simulink model "North_Country_Grid_2024a"  (R2024a)
settings: Solver=VariableStepAuto  StartTime=0.0  StopTime=10  RelTol=1e-3
PreLoadFcn:
  | Ts=50e-6;
InitFcn:
  | xInitial = WindFarmType4AverageModelInit;
  | Ts=50e-6;
undefined symbols (not defined in the file or in its folder): D1, D11, Delta, DiscIntNeverNeededParam, find_system, Fnom_I, Fnom_R, Idc_nom, lagging, level, pulse, test_alpha, Vdc_nom, VLL_nom_I, VLL_nom_R
libraries: spsSecondOrderFilterLib x47, powerlib_extras x38, simulink x34, spsThreePhaseVIMeasurementLib x30, spsFirstOrderFilterLib x29, simulink_extras x26, spsabctodq0Lib x25, spsThreePhaseTransformerTwoWindingsLib x19, spsThreePhaseBreakerLib x18, spsThreePhasePISectionLineLib x17, spsControlledVoltageSourceLib x15, spsOnDelayLib x12
(part 1 of 18)
settings Model: FPTRunName=Active  Creator=The MathWorks, Inc.  LastModifiedBy=prankfarsons
settings DebuggingCC: UnderspecifiedInitializationDetection=Classic  MergeDetectMultiDrivingBlocksExec=none
settings ModelReferenceCC: PropagateSignalLabelsOutOfModel=off

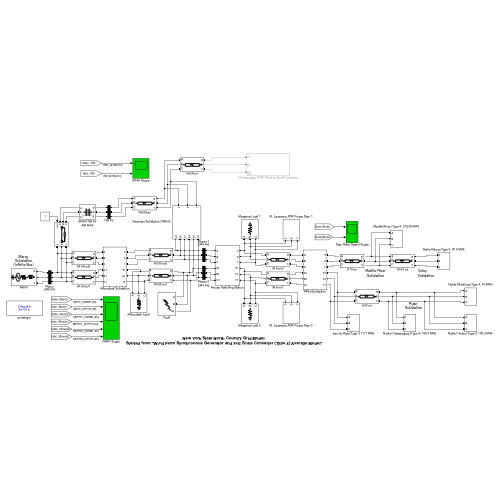
[thumbnail: Simulink's stored preview of the top-level diagram]
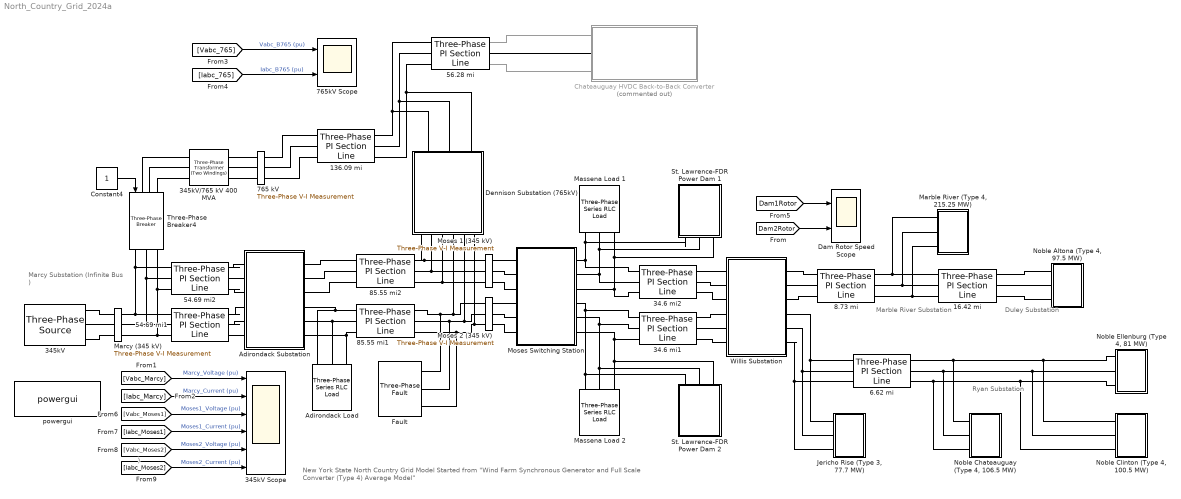
== system North_Country_Grid_2024a ==
  note: )
  note: Marcy Substation
      | (Infinite Bus )
  note: Ryan Substation
  note: New York State North Country Grid Model
      | Started from "Wind Farm Synchronous Generator and Full Scale Converter (Type 4) Average Model"
  note: Marble River Substation
  note: Duley Substation
  " Dam Rotor Speed Scope" : Scope  NumInputPorts=2
  136.09 mi : spsThreePhasePISectionLineLib/Three-Phase PI Section Line  LConnTagsString=a|b|c  RConnTagsString=A|B|C  Length=219.015  Frequency=60  Resistances=[0.0117 0.3864]  Inductances="[9.44e-4  4.1264e-3]"  Capacitances=[4e-10 7.751e-9]
  16.42 mi : spsThreePhasePISectionLineLib/Three-Phase PI Section Line  LConnTagsString=a|b|c  RConnTagsString=A|B|C  Length=26.425  Frequency=60  Resistances=[ 0.0283 0.3864]  Inductances="[ 1.146e-3  4.1264e-3]"  Capacitances=[20.9e-9 7.751e-9]
  34.6 mi1 : spsThreePhasePISectionLineLib/Three-Phase PI Section Line  LConnTagsString=a|b|c  RConnTagsString=A|B|C  Length=55.68  Frequency=60  Resistances=[ 0.0283 0.3864]  Inductances="[ 1.146e-3  4.1264e-3]"  Capacitances=[20.9e-9 7.751e-9]
  34.6 mi2 : spsThreePhasePISectionLineLib/Three-Phase PI Section Line  LConnTagsString=a|b|c  RConnTagsString=A|B|C  Length=55.68  Frequency=60  Resistances=[ 0.0283 0.3864]  Inductances="[ 1.146e-3  4.1264e-3]"  Capacitances=[20.9e-9 7.751e-9]
  345kV : spsThreePhaseSourceLib/Three-Phase Source  InternalConnection=Yg  VoltagePhases=off  Voltage=(345000)*0.996321  PhaseAngle=0.044565  Voltage_phases=[25e3 25e3 25e3]/sqrt(3)  PhaseAngles_phases=[0 -120 +120]  Frequency=60  NonIdealSource=on  SpecifyImpedance=off  Resistance=0.8929  Inductance=16.58e-3  ShortCircuitLevel=100e6  BaseVoltage=345e3  XRratio=7  BusType=swing  Pref=100000000  Qref=0  Prefabc=[10e3, 10e3, 10e3]  Qrefabc=[0, 0, 0]  Qmin=-Inf  Qmax=Inf
  345kV Scope : Scope  NumInputPorts=6
  345kV/765 kV 400 MVA : spsThreePhaseTransformerTwoWindingsLib/Three-Phase Transformer (Two Windings)  Winding1Connection=Delta (D11)  Winding2Connection=Yg  CoreType=Three single-phase transformers  SetSaturation=off  Hysteresis=off  DataFile='basic_model'  SetInitialFlux=off  Measurements=None  UNITS=pu  NominalPower=[400e6 60 ]  Winding1="[ 345e3  0.0125   0.025 ]"  Winding2="[765e3  0.0125   0.025]"  Rm=500  Lm=inf  L0=0.5  Saturation="[ 0,0  ;  0.005,1.2  ;  1.0,1.4 ]"  InitialFluxes=[ 0.8 , -0.8 , 0.7 ]  BreakLoop=off  DiscreteSolver=Trapezoidal iterative  DataType=off  TransfoNumber=0
  54.69 mi1 : spsThreePhasePISectionLineLib/Three-Phase PI Section Line  LConnTagsString=a|b|c  RConnTagsString=A|B|C  Length=88.015  Frequency=60  Resistances=[ 0.0283 0.3864]  Inductances="[ 1.146e-3  4.1264e-3]"  Capacitances=[20.9e-9 7.751e-9]
  54.69 mi2 : spsThreePhasePISectionLineLib/Three-Phase PI Section Line  LConnTagsString=a|b|c  RConnTagsString=A|B|C  Length=88.015  Frequency=60  Resistances=[ 0.0283 0.3864]  Inductances="[ 1.146e-3  4.1264e-3]"  Capacitances=[20.9e-9 7.751e-9]
  56.28 mi : spsThreePhasePISectionLineLib/Three-Phase PI Section Line  LConnTagsString=a|b|c  RConnTagsString=A|B|C  Length=90.57  Frequency=60  Resistances=[0.0117 0.3864]  Inductances="[9.44e-4  4.1264e-3]"  Capacitances=[4e-10 7.751e-9]
  6.62 mi : spsThreePhasePISectionLineLib/Three-Phase PI Section Line  LConnTagsString=a|b|c  RConnTagsString=A|B|C  Length=10.654  Frequency=60  Resistances=[ 0.0283 0.3864]  Inductances="[ 1.146e-3  4.1264e-3]"  Capacitances=[20.9e-9 7.751e-9]
  765 kV : spsThreePhaseVIMeasurementLib/Three-Phase V-I Measurement  VoltageMeasurement=phase-to-ground  SetLabelV=on  LabelV=Vabc_765  Vpu=on  VpuLL=off  CurrentMeasurement=yes  SetLabelI=on  LabelI=Iabc_765  Ipu=on  Pbase=1590.45e6  Vbase=765e3  OutputType=Complex  PhasorSimulation=off  PSBequivalent=0
  765kV Scope : Scope  NumInputPorts=2
  8.73 mi : spsThreePhasePISectionLineLib/Three-Phase PI Section Line  LConnTagsString=a|b|c  RConnTagsString=A|B|C  Length=14.049  Frequency=60  Resistances=[ 0.0283 0.3864]  Inductances="[ 1.146e-3  4.1264e-3]"  Capacitances=[20.9e-9 7.751e-9]
  85.55 mi1 : spsThreePhasePISectionLineLib/Three-Phase PI Section Line  LConnTagsString=a|b|c  RConnTagsString=A|B|C  Length=137.679  Frequency=60  Resistances=[ 0.0283 0.3864]  Inductances="[ 1.146e-3  4.1264e-3]"  Capacitances=[20.9e-9 7.751e-9]
  85.55 mi2 : spsThreePhasePISectionLineLib/Three-Phase PI Section Line  LConnTagsString=a|b|c  RConnTagsString=A|B|C  Length=137.679  Frequency=60  Resistances=[ 0.0283 0.3864]  Inductances="[ 1.146e-3  4.1264e-3]"  Capacitances=[20.9e-9 7.751e-9]
  Adirondack Load : spsThreePhaseSeriesRLCLoadLib/Three-Phase Series RLC Load  LConnTagsString=A|B|C  Configuration=Y (grounded)  NominalVoltage=345e3  Vabc=[1e3 1e3 1e3]  Vabcp=[1e3 1e3 1e3]  NominalFrequency=60  UnbalancedPower=off  ActivePower=100000000  InductivePower=0  CapacitivePower=0  Pabc=[10e3 9e3 11e3]  QLabc=[100 90 110]  QCabc=[100 90 110]  Pabcp=[10e3 9e3 11e3]  QLabcp=[100 90 110]  QCabcp=[100 90 110]  Measurements=None  LoadType=constant Z
  Adirondack Substation : Subsystem
  Chateauguay HVDC Back-to-Back Converter : Subsystem  Commented=on
  Constant4 : Constant
  Dennison Substation (765kV) : Subsystem
      settings: PortSchema="{\"entries\":[{\"content\":{\"sides\":[{\"content\":{},\"type\":\"ConnectorPlacement.EquallySpacedRectSide\",\"uuid\":\"bf43bd2c-e3a2-40b5-9bf7-800fca43b76b\"},{\"content\":{\"side\":\"RIGHT\"},\"type\":\"ConnectorPlacement.EquallySpacedRectSide\",\"uuid\":\"0e930517-6b8c-4af0-8fde-37d9fd24c178\"},{\"content\":{\"connectorIds\":[\"LConn1\",\"LConn2\",\"LConn3\"],\"side\":\"TOP\"},\"type\":\"ConnectorPlacement.EquallySpacedRectSide\",\"uuid\":\"782c9b1f-adb6-4d18-a320-946579c28cc2\"},{\"content\":{\"connectorIds\":[\"RConn1\",\"RConn2\",\"RConn3\",\"RConn4\",\"RConn5\",\"RConn6\"],\"side\":\"BOTTOM\"},\"type\":\"ConnectorPlacement.EquallySpacedRectSide\",\"uuid\":\"c85884d3-7f69-4181-84c4-a6d381e135a3\"}]},\"type\":\"ConnectorPlacement.EquallySpacedConnector\",\"uuid\":\"dcc53c74-8f9c-434c-bbfe-404556b3529c\"}],\"packageUris\":[\"http://schema.mathworks.com/mf0/Connector/R2020b\"],\"version\":\"1.0\"}"
  Fault : spsThreePhaseFaultLib/Three-Phase Fault  InitialStates=0  FaultA=on  FaultB=on  FaultC=on  GroundFault=on  SwitchTimes="[4  4.3]"  External=off  SwitchStatus=NaN  FaultResistance=0.001  GroundResistance=0.01  SnubberResistance=1e6  SnubberCapacitance=inf  Measurements=None
  "Jericho Rise (Type 3, 77.7 MW)" : Subsystem
  "Marble River (Type 4, 215.25 MW)" : Subsystem
  Marcy (345 kV) : spsThreePhaseVIMeasurementLib/Three-Phase V-I Measurement  VoltageMeasurement=phase-to-ground  SetLabelV=on  LabelV=Vabc_Marcy  Vpu=on  VpuLL=off  CurrentMeasurement=yes  SetLabelI=on  LabelI=Iabc_Marcy  Ipu=on  Pbase=648.45e6  Vbase=345e3  OutputType=Complex  PhasorSimulation=off  PSBequivalent=0
  Massena Load 1 : spsThreePhaseSeriesRLCLoadLib/Three-Phase Series RLC Load  LConnTagsString=A|B|C  Configuration=Y (grounded)  NominalVoltage=345e3  Vabc=[1e3 1e3 1e3]  Vabcp=[1e3 1e3 1e3]  NominalFrequency=60  UnbalancedPower=off  ActivePower=150000000  InductivePower=0  CapacitivePower=0  Pabc=[10e3 9e3 11e3]  QLabc=[100 90 110]  QCabc=[100 90 110]  Pabcp=[10e3 9e3 11e3]  QLabcp=[100 90 110]  QCabcp=[100 90 110]  Measurements=None  LoadType=constant Z
  Massena Load 2 : spsThreePhaseSeriesRLCLoadLib/Three-Phase Series RLC Load  LConnTagsString=A|B|C  Configuration=Y (grounded)  NominalVoltage=345e3  Vabc=[1e3 1e3 1e3]  Vabcp=[1e3 1e3 1e3]  NominalFrequency=60  UnbalancedPower=off  ActivePower=150000000  InductivePower=0  CapacitivePower=0  Pabc=[10e3 9e3 11e3]  QLabc=[100 90 110]  QCabc=[100 90 110]  Pabcp=[10e3 9e3 11e3]  QLabcp=[100 90 110]  QCabcp=[100 90 110]  Measurements=None  LoadType=constant Z
  Moses 1 (345 kV) : spsThreePhaseVIMeasurementLib/Three-Phase V-I Measurement  VoltageMeasurement=phase-to-ground  SetLabelV=on  LabelV=Vabc_Moses1  Vpu=on  VpuLL=off  CurrentMeasurement=yes  SetLabelI=on  LabelI=Iabc_Moses1  Ipu=on  Pbase=648.45e6  Vbase=345e3  OutputType=Complex  PhasorSimulation=off  PSBequivalent=0
  Moses 2 (345 kV) : spsThreePhaseVIMeasurementLib/Three-Phase V-I Measurement  VoltageMeasurement=phase-to-ground  SetLabelV=on  LabelV=Vabc_Moses2  Vpu=on  VpuLL=off  CurrentMeasurement=yes  SetLabelI=on  LabelI=Iabc_Moses2  Ipu=on  Pbase=648.45e6  Vbase=345e3  OutputType=Complex  PhasorSimulation=off  PSBequivalent=0
  Moses Switching Station : Subsystem
  "Noble Altona (Type 4, 97.5 MW)" : Subsystem
  "Noble Chateauguay (Type 4, 106.5 MW)" : Subsystem
  "Noble Clinton (Type 4, 100.5 MW)" : Subsystem
  "Noble Ellenburg (Type 4, 81 MW)" : Subsystem
  St. Lawrence-FDR Power Dam 1 : Subsystem
  St. Lawrence-FDR Power Dam 2 : Subsystem
  Three-Phase Breaker4 : spsThreePhaseBreakerLib/Three-Phase Breaker  InitialState=closed  SwitchA=on  SwitchB=on  SwitchC=on  SwitchTimes="[1/60  5/60]"  External=on  BreakerResistance=0.01  SnubberResistance=1e6  SnubberCapacitance=inf  Measurements=None
  Willis Substation : Subsystem
  powergui : spspowerguiLib/powergui  SimulationMode=Discrete  SampleTime=Ts  frequency=60  Iterations=50  frequencyindice=0  Pbase=100e6  ErrMax=1e-4  UnitsV=kV  UnitsW=MW  buscounter=0  FunctionMessages=off  echomessages=off  EnableUseOfTLC=off  CurrentSourceSwitches=off  DisableSnubberDevices=off  DisableRonSwitches=off  DisableVfSwitches=off  DisplayEquations=off  AutomaticDiscreteSolvers=off  SolverType=Tustin/Backward Euler (TBE)  Interpol=off  ExternalGateDelay=off  methode=off  Ts=0  x0status=blocks  SPID=off  SwTol=0  HookPort=off  NonlinearTolerance=1e-4  nMaxIteration=100  ContinueOnMaxIteration=off  RestoreLinks=warning  ResistiveCurrentMeasurement=off  Frange=[0:2:500]  Ylog=off  Xlog=on  ShowGrid=off  save=off  variable=ZData  structure=0  ZoomFFT=on  StartTime=0.0  cycles=1  DisplayStyle=1  fundamental=60  FreqAxis=off  MaxFrequency=1000  frequencyindicesteady=1  RmsSteady=1  display=off
  wires:
  [Vabc_Marcy] -> 345kV Scope/1  "Marcy_Voltage (pu)"
  [Iabc_Marcy] -> 345kV Scope/2  "Marcy_Current (pu)"
  Constant4/1 -> Three-Phase Breaker4/1
  [Vabc_765] -> 765kV Scope/1  "Vabc_B765 (pu)"
  [Iabc_765] -> 765kV Scope/2  "Iabc_B765 (pu)"
  [Dam2Rotor] -> " Dam Rotor Speed Scope"/2
  [Dam1Rotor] -> " Dam Rotor Speed Scope"/1
  [Vabc_Moses1] -> 345kV Scope/3  "Moses1_Voltage (pu)"
  [Iabc_Moses1] -> 345kV Scope/4  "Moses1_Current (pu)"
  [Vabc_Moses2] -> 345kV Scope/5  "Moses2_Voltage (pu)"
  [Iabc_Moses2] -> 345kV Scope/6  "Moses2_Current (pu)"
  connections:
  16.42 mi/RConn1 -- "Noble Altona (Type 4, 97.5 MW)"/LConn1
  16.42 mi/RConn2 -- "Noble Altona (Type 4, 97.5 MW)"/LConn2
  16.42 mi/RConn3 -- "Noble Altona (Type 4, 97.5 MW)"/LConn3
  8.73 mi/RConn1 -- "Marble River (Type 4, 215.25 MW)"/LConn1 -- 16.42 mi/LConn1
  8.73 mi/RConn2 -- "Marble River (Type 4, 215.25 MW)"/LConn2 -- 16.42 mi/LConn2
  8.73 mi/RConn3 -- "Marble River (Type 4, 215.25 MW)"/LConn3 -- 16.42 mi/LConn3
  "Noble Chateauguay (Type 4, 106.5 MW)"/LConn1 -- 6.62 mi/RConn1 -- "Noble Ellenburg (Type 4, 81 MW)"/LConn1 -- "Noble Clinton (Type 4, 100.5 MW)"/LConn1
  "Noble Chateauguay (Type 4, 106.5 MW)"/LConn2 -- 6.62 mi/RConn2 -- "Noble Ellenburg (Type 4, 81 MW)"/LConn2 -- "Noble Clinton (Type 4, 100.5 MW)"/LConn2
  "Noble Chateauguay (Type 4, 106.5 MW)"/LConn3 -- 6.62 mi/RConn3 -- "Noble Ellenburg (Type 4, 81 MW)"/LConn3 -- "Noble Clinton (Type 4, 100.5 MW)"/LConn3
  Marcy (345 kV)/RConn1 -- Three-Phase Breaker4/RConn1 -- 54.69 mi2/LConn1 -- 54.69 mi1/LConn1
  Marcy (345 kV)/RConn2 -- Three-Phase Breaker4/RConn2 -- 54.69 mi2/LConn2 -- 54.69 mi1/LConn2
  Marcy (345 kV)/RConn3 -- Three-Phase Breaker4/RConn3 -- 54.69 mi2/LConn3 -- 54.69 mi1/LConn3
  Willis Substation/LConn1 -- 34.6 mi2/RConn1
  Willis Substation/RConn1 -- 8.73 mi/LConn1
  Willis Substation/RConn2 -- 8.73 mi/LConn2
  6.62 mi/LConn1 -- "Jericho Rise (Type 3, 77.7 MW)"/LConn1 -- Willis Substation/RConn4
  Willis Substation/RConn5 -- 6.62 mi/LConn2 -- "Jericho Rise (Type 3, 77.7 MW)"/LConn2
  Willis Substation/RConn6 -- 6.62 mi/LConn3 -- "Jericho Rise (Type 3, 77.7 MW)"/LConn3
  Massena Load 1/LConn1 -- 34.6 mi2/LConn1 -- Moses Switching Station/RConn1 -- St. Lawrence-FDR Power Dam 1/LConn1
  Moses Switching Station/RConn2 -- 34.6 mi2/LConn2 -- Massena Load 1/LConn2 -- St. Lawrence-FDR Power Dam 1/LConn2
  Moses Switching Station/RConn3 -- 34.6 mi2/LConn3 -- Massena Load 1/LConn3 -- St. Lawrence-FDR Power Dam 1/LConn3
  Moses Switching Station/RConn4 -- Massena Load 2/LConn1 -- St. Lawrence-FDR Power Dam 2/LConn1 -- 34.6 mi1/LConn1
  Moses Switching Station/RConn5 -- St. Lawrence-FDR Power Dam 2/LConn2 -- Massena Load 2/LConn2 -- 34.6 mi1/LConn2
  34.6 mi1/RConn1 -- Willis Substation/LConn4
  34.6 mi1/RConn2 -- Willis Substation/LConn5
  34.6 mi1/RConn3 -- Willis Substation/LConn6
  85.55 mi2/RConn1 -- Moses 1 (345 kV)/LConn1 -- Dennison Substation (765kV)/RConn1
  85.55 mi2/RConn2 -- Moses 1 (345 kV)/LConn2 -- Dennison Substation (765kV)/RConn2
  85.55 mi2/RConn3 -- Moses 1 (345 kV)/LConn3 -- Dennison Substation (765kV)/RConn3
  85.55 mi1/RConn1 -- Moses 2 (345 kV)/LConn1 -- Dennison Substation (765kV)/RConn4 -- Fault/LConn1
  85.55 mi1/RConn2 -- Moses 2 (345 kV)/LConn2 -- Dennison Substation (765kV)/RConn5 -- Fault/LConn2
  Fault/LConn3 -- Dennison Substation (765kV)/RConn6 -- Moses 2 (345 kV)/LConn3 -- 85.55 mi1/RConn3
  85.55 mi2/LConn1 -- Adirondack Substation/RConn1
  Adirondack Substation/RConn2 -- 85.55 mi2/LConn2
  Adirondack Substation/RConn3 -- 85.55 mi2/LConn3
  Adirondack Substation/RConn4 -- Adirondack Load/LConn1 -- 85.55 mi1/LConn1
  Adirondack Substation/RConn5 -- 85.55 mi1/LConn2 -- Adirondack Load/LConn2
  Adirondack Substation/RConn6 -- 85.55 mi1/LConn3 -- Adirondack Load/LConn3
  54.69 mi2/RConn2 -- Adirondack Substation/LConn2
  54.69 mi2/RConn1 -- Adirondack Substation/LConn1
  54.69 mi2/RConn3 -- Adirondack Substation/LConn3
  54.69 mi1/RConn1 -- Adirondack Substation/LConn4
  54.69 mi1/RConn2 -- Adirondack Substation/LConn5
  54.69 mi1/RConn3 -- Adirondack Substation/LConn6
  345kV/RConn1 -- Marcy (345 kV)/LConn1
  345kV/RConn2 -- Marcy (345 kV)/LConn2
  345kV/RConn3 -- Marcy (345 kV)/LConn3
  Moses Switching Station/RConn6 -- Massena Load 2/LConn3 -- St. Lawrence-FDR Power Dam 2/LConn3 -- 34.6 mi1/LConn3
  56.28 mi/LConn1 -- Dennison Substation (765kV)/LConn1 -- 136.09 mi/RConn1
  56.28 mi/LConn2 -- Dennison Substation (765kV)/LConn2 -- 136.09 mi/RConn2
  56.28 mi/LConn3 -- Dennison Substation (765kV)/LConn3 -- 136.09 mi/RConn3
  765 kV/RConn1 -- 136.09 mi/LConn1
  765 kV/RConn2 -- 136.09 mi/LConn2
  765 kV/RConn3 -- 136.09 mi/LConn3
  345kV/765 kV 400 MVA/RConn1 -- 765 kV/LConn1
  345kV/765 kV 400 MVA/RConn2 -- 765 kV/LConn2
  345kV/765 kV 400 MVA/RConn3 -- 765 kV/LConn3
  Chateauguay HVDC Back-to-Back Converter/LConn1 -- 56.28 mi/RConn1
  Chateauguay HVDC Back-to-Back Converter/LConn3 -- 56.28 mi/RConn3
  34.6 mi2/RConn2 -- Willis Substation/LConn2
  34.6 mi2/RConn3 -- Willis Substation/LConn3
  Willis Substation/RConn3 -- 8.73 mi/LConn3
  56.28 mi/RConn2 -- Chateauguay HVDC Back-to-Back Converter/LConn2
  345kV/765 kV 400 MVA/LConn1 -- Three-Phase Breaker4/LConn1
  345kV/765 kV 400 MVA/LConn2 -- Three-Phase Breaker4/LConn2
  345kV/765 kV 400 MVA/LConn3 -- Three-Phase Breaker4/LConn3
  Moses 1 (345 kV)/RConn2 -- Moses Switching Station/LConn2
  Moses 1 (345 kV)/RConn1 -- Moses Switching Station/LConn1
  Moses 1 (345 kV)/RConn3 -- Moses Switching Station/LConn3
  Moses 2 (345 kV)/RConn1 -- Moses Switching Station/LConn4
  Moses 2 (345 kV)/RConn2 -- Moses Switching Station/LConn5
  Moses 2 (345 kV)/RConn3 -- Moses Switching Station/LConn6

== system North_Country_Grid_2024a/Adirondack Substation ==
  Constant{,1..4} (5 alike) : Constant
  Three-Phase Breaker{,1..4} (5 alike) : spsThreePhaseBreakerLib/Three-Phase Breaker  InitialState=closed  SwitchA=on  SwitchB=on  SwitchC=on  SwitchTimes="[1/60  5/60]"  External=on  BreakerResistance=0.01  SnubberResistance=1e6  SnubberCapacitance=inf  Measurements=None
  a : PMIOPort  Side=Right
  A : PMIOPort  Port=2  Side=Left
  B : PMIOPort  Port=3  Side=Left
  b : PMIOPort  Port=4  Side=Right
  C : PMIOPort  Port=5  Side=Left
  c : PMIOPort  Port=6  Side=Right
  a1 : PMIOPort  Port=7  Side=Right
  A1 : PMIOPort  Port=8  Side=Left
  b1 : PMIOPort  Port=9  Side=Right
  B1 : PMIOPort  Port=10  Side=Left
  C1 : PMIOPort  Port=11  Side=Left
  c1 : PMIOPort  Port=12  Side=Right
  wires:
  Constant/1 -> Three-Phase Breaker/1
  Constant2/1 -> Three-Phase Breaker2/1
  Constant1/1 -> Three-Phase Breaker1/1
  Constant4/1 -> Three-Phase Breaker4/1
  Constant3/1 -> Three-Phase Breaker3/1
  connections:
  Three-Phase Breaker1/LConn3 -- C/RConn1
  Three-Phase Breaker1/LConn1 -- A/RConn1
  Three-Phase Breaker2/LConn1 -- A1/RConn1
  Three-Phase Breaker/RConn3 -- c/RConn1
  Three-Phase Breaker3/RConn3 -- c1/RConn1
  Three-Phase Breaker/RConn2 -- b/RConn1
  Three-Phase Breaker1/LConn2 -- B/RConn1
  Three-Phase Breaker/LConn2 -- Three-Phase Breaker1/RConn2 -- Three-Phase Breaker4/LConn2
  Three-Phase Breaker2/RConn3 -- Three-Phase Breaker4/RConn3 -- Three-Phase Breaker3/LConn3
  Three-Phase Breaker2/LConn3 -- C1/RConn1
  Three-Phase Breaker/RConn1 -- a/RConn1
  Three-Phase Breaker3/LConn1 -- Three-Phase Breaker2/RConn1 -- Three-Phase Breaker4/RConn1
  Three-Phase Breaker3/RConn2 -- b1/RConn1
  Three-Phase Breaker2/RConn2 -- Three-Phase Breaker3/LConn2 -- Three-Phase Breaker4/RConn2
  Three-Phase Breaker4/LConn3 -- Three-Phase Breaker1/RConn3 -- Three-Phase Breaker/LConn3
  Three-Phase Breaker2/LConn2 -- B1/RConn1
  Three-Phase Breaker3/RConn1 -- a1/RConn1
  Three-Phase Breaker4/LConn1 -- Three-Phase Breaker1/RConn1 -- Three-Phase Breaker/LConn1

== system North_Country_Grid_2024a/Chateauguay HVDC Back-to-Back Converter ==
  note: 345kV, 60 Hz,
      | 10,000 MVA equivalent
  note: phi = 80 deg. 3rd harm.
  " 50 Hz 345kV  " : spsThreePhaseSourceLib/Three-Phase Source  InternalConnection=Yg  VoltagePhases=off  Voltage=VLL_nom_I  PhaseAngle=0  Voltage_phases=[25e3 25e3 25e3]/sqrt(3)  PhaseAngles_phases=[0 -120 +120]  Frequency=60  NonIdealSource=on  SpecifyImpedance=off  Resistance=0  Inductance=28.0e-3  ShortCircuitLevel=0  BaseVoltage=0  XRratio=0  BusType=swing  Pref=0  Qref=0  Prefabc=[10e3, 10e3, 10e3]  Qrefabc=[0, 0, 0]  Qmin=-inf  Qmax=inf
  0.5 H : spsSeriesRLCBranchLib/Series RLC Branch  LConnTagsString=__new0  RConnTagsString=__new0  BranchType=RL  Resistance=1  Inductance=0.5  SetiL0=off  InitialCurrent=0  Capacitance=1.0  Setx0=off  InitialVoltage=0  Measurements=None
  "0.5 H " : spsSeriesRLCBranchLib/Series RLC Branch  LConnTagsString=__new0  RConnTagsString=__new0  BranchType=RL  Resistance=1  Inductance=0.5  SetiL0=off  InitialCurrent=0  Capacitance=1.0  Setx0=off  InitialVoltage=0  Measurements=None
  3- Phase Parallel RLC1 : spsThreePhaseParallelRLCBranchLib/Three-Phase Parallel RLC Branch  LConnTagsString=A|B|C  RConnTagsString=A|B|C  BranchType=RL  Resistance=6.205  Inductance=13.96e-3  Capacitance=1.0  Measurements=None
  Binv : spsThreePhaseVIMeasurementLib/Three-Phase V-I Measurement  VoltageMeasurement=phase-to-ground  SetLabelV=on  LabelV=Vabc_I  Vpu=on  VpuLL=off  CurrentMeasurement=yes  SetLabelI=on  LabelI=Iabc_I  Ipu=on  Pbase=100e6  Vbase=345e3  OutputType=Magnitude  PhasorSimulation=off  PSBequivalent=0
  Brect : spsThreePhaseVIMeasurementLib/Three-Phase V-I Measurement  VoltageMeasurement=phase-to-ground  SetLabelV=on  LabelV=Vabc_R  Vpu=on  VpuLL=off  CurrentMeasurement=yes  SetLabelI=on  LabelI=Iabc_R  Ipu=on  Pbase=100e6  Vbase=500e3  OutputType=Magnitude  PhasorSimulation=off  PSBequivalent=0
  Data Acquisition : Subsystem
      mask Display: disp('Open this block\nto visualize\nrecorded signals')
  Ground1 : spsGroundLib/Ground  LConnTagsString=a
  Ground4 : spsGroundLib/Ground  LConnTagsString=a
  Inverter : Subsystem
  Inverter Control and Protection : Subsystem
      mask Display: disp('Pole Control\n and Protection')
  Master Control : Subsystem
      mask Display: disp('Master Control')
  Rectifier : Subsystem
  Rectifier Control and Protection : Subsystem
      mask Display: disp('Pole Control\n and Protection')
  A : PMIOPort  Side=Left
  B : PMIOPort  Port=2  Side=Left
  C : PMIOPort  Port=3  Side=Left
  connections:
  0.5 H/RConn1 -- "0.5 H "/RConn1
  Brect/RConn2 -- Rectifier/LConn2
  Brect/RConn3 -- Rectifier/LConn3
  "0.5 H "/LConn1 -- Inverter/RConn1
  Inverter/LConn1 -- Binv/RConn1
  Ground1/LConn1 -- Inverter/RConn2
  Inverter/LConn3 -- Binv/RConn3
  Rectifier/RConn2 -- Ground4/LConn1
  Brect/RConn1 -- Rectifier/LConn1
  3- Phase Parallel RLC1/LConn3 -- " 50 Hz 345kV  "/RConn3
  3- Phase Parallel RLC1/LConn1 -- " 50 Hz 345kV  "/RConn1
  3- Phase Parallel RLC1/LConn2 -- " 50 Hz 345kV  "/RConn2
  Inverter/LConn2 -- Binv/RConn2
  0.5 H/LConn1 -- Rectifier/RConn1
  Binv/LConn1 -- A/RConn1
  Binv/LConn2 -- B/RConn1
  Binv/LConn3 -- C/RConn1
  3- Phase Parallel RLC1/RConn1 -- Brect/LConn1
  3- Phase Parallel RLC1/RConn2 -- Brect/LConn2
  3- Phase Parallel RLC1/RConn3 -- Brect/LConn3

== system North_Country_Grid_2024a/Dennison Substation (765kV) ==
  345kV/765 kV 400 MVA1 : spsThreePhaseTransformerTwoWindingsLib/Three-Phase Transformer (Two Windings)  Winding1Connection=Delta (D11)  Winding2Connection=Yg  CoreType=Three single-phase transformers  SetSaturation=off  Hysteresis=off  DataFile='basic_model'  SetInitialFlux=off  Measurements=None  UNITS=pu  NominalPower=[400e6 60 ]  Winding1="[ 345e3  0.0125   0.025 ]"  Winding2="[765e3  0.0125   0.025]"  Rm=500  Lm=inf  L0=0.5  Saturation="[ 0,0  ;  0.005,1.2  ;  1.0,1.4 ]"  InitialFluxes=[ 0.8 , -0.8 , 0.7 ]  BreakLoop=off  DiscreteSolver=Trapezoidal iterative  DataType=off  TransfoNumber=0
  345kV/765 kV 400 MVA2 : spsThreePhaseTransformerTwoWindingsLib/Three-Phase Transformer (Two Windings)  Winding1Connection=Delta (D11)  Winding2Connection=Yg  CoreType=Three single-phase transformers  SetSaturation=off  Hysteresis=off  DataFile='basic_model'  SetInitialFlux=off  Measurements=None  UNITS=pu  NominalPower=[400e6 60 ]  Winding1="[ 345e3  0.0125   0.025 ]"  Winding2="[765e3  0.00025   0.0125   0.025]"  Rm=500  Lm=inf  L0=0.5  Saturation="[ 0,0  ;  0.005,1.2  ;  1.0,1.4 ]"  InitialFluxes=[ 0.8 , -0.8 , 0.7 ]  BreakLoop=off  DiscreteSolver=Trapezoidal iterative  DataType=off  TransfoNumber=0
  Constant1 : Constant
  Constant2 : Constant
  Three-Phase Breaker1 : spsThreePhaseBreakerLib/Three-Phase Breaker  InitialState=closed  SwitchA=on  SwitchB=on  SwitchC=on  SwitchTimes="[1/60  5/60]"  External=on  BreakerResistance=0.01  SnubberResistance=1e6  SnubberCapacitance=inf  Measurements=None
  Three-Phase Breaker2 : spsThreePhaseBreakerLib/Three-Phase Breaker  InitialState=closed  SwitchA=on  SwitchB=on  SwitchC=on  SwitchTimes="[1/60  5/60]"  External=on  BreakerResistance=0.01  SnubberResistance=1e6  SnubberCapacitance=inf  Measurements=None
  a : PMIOPort  Side=Left
  b : PMIOPort  Port=2  Side=Left
  c : PMIOPort  Port=3  Side=Left
  a2 : PMIOPort  Port=4  Side=Right
  b2 : PMIOPort  Port=5  Side=Right
  c2 : PMIOPort  Port=6  Side=Right
  a3 : PMIOPort  Port=7  Side=Right
  b3 : PMIOPort  Port=8  Side=Right
  c3 : PMIOPort  Port=9  Side=Right
  wires:
  Constant1/1 -> Three-Phase Breaker1/1
  Constant2/1 -> Three-Phase Breaker2/1
  connections:
  345kV/765 kV 400 MVA2/RConn3 -- c/RConn1 -- 345kV/765 kV 400 MVA1/RConn3
  345kV/765 kV 400 MVA2/RConn1 -- 345kV/765 kV 400 MVA1/RConn1 -- a/RConn1
  345kV/765 kV 400 MVA2/RConn2 -- 345kV/765 kV 400 MVA1/RConn2 -- b/RConn1
  345kV/765 kV 400 MVA1/LConn1 -- Three-Phase Breaker1/LConn1
  345kV/765 kV 400 MVA1/LConn2 -- Three-Phase Breaker1/LConn2
  345kV/765 kV 400 MVA1/LConn3 -- Three-Phase Breaker1/LConn3
  345kV/765 kV 400 MVA2/LConn1 -- Three-Phase Breaker2/LConn1
  345kV/765 kV 400 MVA2/LConn2 -- Three-Phase Breaker2/LConn2
  345kV/765 kV 400 MVA2/LConn3 -- Three-Phase Breaker2/LConn3
  a2/RConn1 -- Three-Phase Breaker1/RConn1
  b2/RConn1 -- Three-Phase Breaker1/RConn2
  c2/RConn1 -- Three-Phase Breaker1/RConn3
  c3/RConn1 -- Three-Phase Breaker2/RConn3
  b3/RConn1 -- Three-Phase Breaker2/RConn2
  a3/RConn1 -- Three-Phase Breaker2/RConn1

== system North_Country_Grid_2024a/Jericho Rise (Type 3, 77.7 MW) ==
  1 km collector line : spsThreePhasePISectionLineLib/Three-Phase PI Section Line  LConnTagsString=a|b|c  RConnTagsString=A|B|C  Length=1  Frequency=60  Resistances=[ 0.01273 0.3864]  Inductances="[ 0.9337e-3  4.1264e-3]"  Capacitances=[12.74e-9 7.751e-9]
  115 kV/34.5 kV 400 MVA : spsThreePhaseTransformerTwoWindingsLib/Three-Phase Transformer (Two Windings)  Winding1Connection=Yg  Winding2Connection=Delta (D11)  CoreType=Three single-phase transformers  SetSaturation=off  Hysteresis=off  DataFile='basic_model'  SetInitialFlux=off  Measurements=None  UNITS=pu  NominalPower=[400e6 60 ]  Winding1="[ 115e3  0.0125   0.025 ]"  Winding2="[34.5e3  0.0125  0.025]"  Rm=500  Lm=500  L0=0.5  Saturation="[ 0,0  ;  0.005,1.2  ;  1.0,1.4 ]"  InitialFluxes=[ 0.8 , -0.8 , 0.7 ]  BreakLoop=off  DiscreteSolver=Trapezoidal iterative  DataType=off  TransfoNumber=0
  34.5 kV/ 690V 400 MVA : spsThreePhaseTransformerTwoWindingsLib/Three-Phase Transformer (Two Windings)  Winding1Connection=Delta (D11)  Winding2Connection=Yg  CoreType=Three single-phase transformers  SetSaturation=off  Hysteresis=off  DataFile='hysteresis'  SetInitialFlux=off  Measurements=None  UNITS=pu  NominalPower="[400e6  60]"  Winding1=[34.5e3 , 0.0125 , 0.025]  Winding2=[690, 0.0125, 0.025]  Rm=500  Lm=inf  L0=0.5  Saturation=[ 0,0 ; 0.0024,1.2 ; 1.0,1.52 ]  InitialFluxes=[ 0.8 , -0.8 , 0.7 ]  BreakLoop=off  DiscreteSolver=Trapezoidal iterative  DataType=off  TransfoNumber=0
  345kV/115 kV 400 MVA : spsThreePhaseTransformerTwoWindingsLib/Three-Phase Transformer (Two Windings)  Winding1Connection=Delta (D11)  Winding2Connection=Yg  CoreType=Three single-phase transformers  SetSaturation=off  Hysteresis=off  DataFile='basic_model'  SetInitialFlux=off  Measurements=None  UNITS=pu  NominalPower=[400e6 60 ]  Winding1="[ 345e3  0.0125   0.025 ]"  Winding2="[115e3  0.0125  0.025]"  Rm=500  Lm=inf  L0=0.5  Saturation="[ 0,0  ;  0.005,1.2  ;  1.0,1.4 ]"  InitialFluxes=[ 0.8 , -0.8 , 0.7 ]  BreakLoop=off  DiscreteSolver=Trapezoidal iterative  DataType=off  TransfoNumber=0
  Bus Selector : BusSelector  OutputSignals=Vdc_V,wr_pu (IG speed),PQ_pu.P_pu,PQ_pu.Q_pu
  Constant2 : Constant  Value=15
  Constant3 : Constant  Value=0
  DFIG Wind Turbine : Subsystem  LoadFcn=%find_system(gcs,'FollowLinks', 'on', 'LookUnderMasks', 'all');  mask(DFIG Wind Turbine){Nb_wt=37, ShowParameters=Control parameters for 1 wind turbine, nom=[2.1e6 690 845 60], sta=[ 0.023 0.18], rot=[ 0.016 0.16], Lm=2.9, mec=[0.685 0.01 3], init=[ -0.2,0   0,0,0   0,0,0 ], Imax_grid_conv=0.8, RL_grid=[ 0.3 0.003], Vdc_nom=1150, C_DClink1=10000e-6, C_var_filter1=120e3, Pmec1=1.5e6, wind_speed_CpMax=11, wind0=11, DisplayTurbChar=off, H_WT=4.32, Ksh=1.11, D_mutual=1.5, w_wt0=1.2, torque0=0.83, Kdc=[8   400], Kgrid_side_cur_reg=[0.83 5], Kspeed=[3 0.6], Krotor_side_cur_reg=[0.6 8], Ki_QV=[0.05 20], Kp_pitch=[150], Kcompensation=[3 30], PWM_freq_grid=2700, PWM_freq_rotor=1620, pitch_max=27, pitch_rate=10}
      mask prompts: Nb_wt "Number of wind turbines:"; ShowParameters "Display:"; nom "Nom. power, L-L volt. and freq. [Pn (VA), Vs_nom (Vrms), Vr_nom (Vrms), fn (Hz)]:"; sta "Stator [ Rs,Lls ] (p.u.):"; rot "Rotor [ Rr',Llr' ] (p.u.):"; Lm "Magnetizing inductance Lm (p.u.):"; mec "Inertia constant, friction factor, and pairs of poles [ H(s)  F(p.u.)  p ]:"; init "Initial conditions [s  th  ias  ibs  ics  phaseas phasebs phasecs]:"; Imax_grid_conv "Grid-side converter maximum current (pu of generator nominal current):"; RL_grid "Grid-side coupling inductor [ L, R] (p.u.):"; Vdc_nom "Nominal DC bus voltage (V):"; C_DClink1 "DC bus capacitor (F):"; C_var_filter1 "Line filter capacitor (Q=50) (var):"; Pmec1 "Nominal mechanical output power (W):"; wind_speed_CpMax "Wind speed at nominal speed and at Cp max (must be between 6 m/s and 30 m/s) (m/s):"; wind0 "Initial wind speed (m/s):"; DisplayTurbChar "Display wind turbine power characteristics:"; H_WT "Wind turbine inertia constant H (s):"; Ksh "Shaft spring constant refer to high-speed shaft (pu of nominal mechanical torque/rad):"; D_mutual "Shaft mutual damping (pu of nominal mechanical torque/pu dw):"; w_wt0 "Turbine initial speed (pu of nominal speed):"; torque0 "Initial output torque (pu of nominal mechanical torque):"; Kdc "DC bus voltage regulator gains [Kp Ki]:"; Kgrid_side_cur_reg "Grid-side converter current regulator gains [Kp Ki]:"; Kspeed "Speed regulator gains [Kp Ki]:"; Krotor_side_cur_reg "Rotor-side converter current regulator gains [Kp Ki]:"; Ki_QV "Q and V regulator gains [Ki_var Ki_volt]:"; Kp_pitch "Pitch controller gain [Kp]:"; Kcompensation "Pitch compensation gains [Kp Ki]:"; PWM_freq_grid "Frequency of the grid-side PWM carrier (Hz):"; PWM_freq_rotor "Frequency of the rotor-side PWM carrier (Hz):"; pitch_max "Maximum pitch angle (deg):"; pitch_rate "Maximum rate of change of pitch angle (deg/s):"
      mask help: This block implements a model of a variable speed pitch controlled wind turbine using a doubly-fed induction generator (DFIG).
      mask init:
      | %Generator data
      | Pnom=nom(1)*Nb_wt;
      | Vnom=nom(2);
      | Vnom_r=nom(3);
      | Fnom=nom(4);
      | Rs=sta(1);
      | Lls=sta(2);
      | Rr=rot(1);
      | Llr=rot(2);
      | H=mec(1);
      | F=mec(2);
      | p=mec(3);
      | 
      | % Converters data
      | L_RL=RL_grid(1);
      | R_RL=RL_grid(2);
      | Q_filter=50;
      | C_DClink=C_DClink1*Nb_wt;
      | C_var_filter=C_var_filter1*Nb_wt;
      | 
      | % Controller data
      | Freq_filter=1000*10;   %Hz
      | Zeta_filter=0.707;
      | Mod_index_max_grid=1.1;   %Maximum value of modulation index for grid-side converter
      | Mod_index_max_rotor=2;   %Maximum value of modulation index for rotor-side converter
      | Lim_grid_side_cur_reg=1.1; %Limit for grid-side PI current regulator (pu)
      | Lim_rotor_side_cur_reg=0.1; %Limit for rotor-side PI current regulator (pu)
      | Min_var_reg=0.9; %Minimum output value for integral var regulator (pu)
      | Max_var_reg=1.1; %Maximum output value for integral var regulator (pu)
      | Max_speed_reg=1; %Maximum output value for PI speed regulator (pu)
      | Kp_dc=Kdc(1);
      | Ki_dc=Kdc(2);
      | Kp_grid_side_cur_reg=Kgrid_side_cur_reg(1);
      | Ki_grid_side_cur_reg=Kgrid_side_cur_reg(2);
      | Kp_speed=Kspeed(1);
      | Ki_speed=Kspeed(2);
      | Kp_compensation=Kcompensation(1);
      | Ki_compensation=Kcompensation(2);
      | Kp_rotor_side_cur_reg=Krotor_side_cur_reg(1);
      | Ki_rotor_side_cur_reg=Krotor_side_cur_reg(2);
      | Ki_var=Ki_QV(1);
      | Ki_volt=Ki_QV(2);
      | Iq_ref_limit_time_constant=0.3; %(s)
      | T_speed=5;      %s
      | Min_mag_flux=0.5;   %(pu)
      | Max_Idr_ref=0.9;    %(pu)
      | Speed_max=1.2;  %(pu)
      | Speed_min=0.7;  %(pu)
      | Pitch_time_constant=0.01;    %(s)
      | 
      | 
      | % Turbine data
      | Pmec=Pmec1*Nb_wt;
      | c1 = 0.6450;
      | c2 = 116;
      | c3 = .4;
      | c4 = 5;
      | c5 = 21;
      | c6 = .00912;  % Set Pmin in stall condition (does not vary with wind_speed_Pmax)
      | c7 = .08;
      | c8 = .035;
      | theta=0;
      | CpMax=.5;
      | lambda_CpMax=9.9495;
      | 
      | c1_c8=[c1 c2 c3 c4 c5 c6 c7 c8];
      |   
      | 
      | %   Cp = c1*(c6*lambda + (-c4 - c3*(2.5 + theta) + c2*(1/(lambda + ...
      | %   c7*(2.5 + theta)) - c8/(1 + (2.5 + theta)^3)))/exp(c5*(1/(lambda + ...
      | %   c7*(2.5 + theta)) - c8/(1 + (2.5 + theta)^3))))
      | 
      | 
      |         %%%%%%%%%%%%%%%%%%%%%%%%%%%%%%%%%%%%%%%%%%%%%%%%%%%%%%%%%%%%%%%%%%%%%%%%%%%
      |         % Operation at Cp max
      |         %%%%%%%%%%%%%%%%%%%%%%%%%%%%%%%%%%%%%%%%%%%%%%%%%%%%%%%%%%%%%%%%%%%%%%%%%%%
      |         
      |         rated_omegar=1.2;
      |         omegar = rated_omegar;
      |         
      |         % Enforce boundaries on wind speed
      |         % A warning could be displayed
      |         if wind_speed_CpMax < 6
      |             wind_speed_CpMax=6;
      |             disp('Warning: Wind speed at nominal speed and at Cp max has been set to 6 m/s')
      |         end
      |         if wind_speed_CpMax > 30
      |             wind_speed_CpMax=30;
      |             disp('Warning: Wind speed at nominal speed and at Cp max has been set to 30 m/s')
      |         end
      | 
      |         K1=lambda_CpMax/omegar*wind_speed_CpMax;
      |         
      |         % Calculation of K2 needed to get P equal to the requested value at
      |         % Cp max for the requested wind speed
      |         
      |         Prated=Pmec1*Nb_wt;
      |         P_rated_omegar_theta_zero=0.75;
      |         
      |         K2 = P_rated_omegar_theta_zero*Prated/(wind_speed_CpMax^3*CpMax);
      |         
      |         K1_K2=[K1 K2];
      |         
      |         %%%%%%%%%%%%%%%%%%%%%%%%%%%%%%%%%%%%%%%%%%%%%%%%%%%%%%%%%%%%%%%%%%%%%%%%%%%
      |         % End of calculation for operation at Cp max
      |         %%%%%%%%%%%%%%%%%%%%%%%%%%%%%%%%%%%%%%%%%%%%%%%%%%%%%%%%%%%%%%%%%%%%%%%%%%%
      |         
      | 
      | %%%%%%%%%%%%%%%%%%%%%%%%%%%%%%%%%%%%%%%%%%%%%%%%%%%%%%%%%%%%%%%%%%%%%%%%%%%
      | % Plot turbine characteristics
      | %%%%%%%%%%%%%%%%%%%%%%%%%%%%%%%%%%%%%%%%%%%%%%%%%%%%%%%%%%%%%%%%%%%%%%%%%%% 
      | 
      | DisplayTurbChar=get_param(gcb,'DisplayTurbChar');
      | if strcmp(DisplayTurbChar,'on')
      |     vect_theta = 0:2:30;
      |     
      |     vect_lambda = 1:0.2:30;
      |     
      |     clear Cp;
      |     
      |     for i=1:length(vect_theta)
      |      for j=1:length(vect_lambda)
      |                 Cp(i,j) = c1*(c6*vect_lambda(j) + (-c4 - c3*(2.5 + vect_theta(i)) + c2*(1/(vect_lambda(j) + ...
      |                 c7*(2.5 + vect_theta(i))) - c8/(1 + (2.5 + vect_theta(i))^3)))/exp(c5*(1/(vect_lambda(j) + ...
      |                 c7*(2.5 + vect_theta(i))) - c8/(1 + (2.5 + vect_theta(i))^3))));
      |      end
      |     end
      | 
      |     figure(1);
      |     clf;
      |     hold on;
      | 
      |     plot(vect_lambda, Cp);
      |     axis([0, 25, 0, .6]);
      |     title('Wind Turbine Cp Characteristic (pitch angle increases by step of 2 deg.)');
      |     ylabel('Cp');
      |     set(gca,'ytick',[0 .1 .2 .3 .4 .5 .6]);
      |     xlabel('Lambda');
      |     grid on;
      |     text(10.1,0.51,'Pitch angle 0 degree');
      | 
      |     hold off
      |     
      |     % Plot of the wind turbine mechanical power output (pu) lambda and Cp
      |     % characteristics against wind speed (m/s) for a range of theta.
      |     
      |     wind_speed_range = [1,.2,30];
      |     vect_wind_speed = 1:0.2:30;
      |     
      |     clear lambda;
      |     clear Cp;
      |     clear P;
      | 
      |     for i=1:length(vect_theta)
      |         for j=1:length(vect_wind_speed)
      |             lambda(i,j) = K1*omegar/vect_wind_speed(j);
      |             Cp(i,j) = c1*(c6*lambda(i,j) + (-c4 - c3*(2.5 + vect_theta(i)) + c2*(1/(lambda(i,j) + ...
      |             c7*(2.5 + vect_theta(i))) - c8/(1 + (2.5 + vect_theta(i))^3)))/exp(c5*(1/(lambda(i,j) + ...
      |             c7*(2.5 + vect_theta(i))) - c8/(1 + (2.5 + vect_theta(i))^3))));
      |             P(i,j) = K2/Prated*vect_wind_speed(j)^3*Cp(i,j);
      |         end
      |     end
      |     
      |     
      |     figure(2);
      |     clf;
      |     hold on
      |     
      |     subplot(3,1,1);
      |     plot(vect_wind_speed, P);
      |     axis([0, 35, 0, 1.5]);
      |     title('Wind Turbine Characteristics (w = 1.2 pu, pitch angle increases by step of 2 deg.)');
      |     ylabel('P (pu)');
      |     set(gca,'ytick',0:.5:4);
      |     grid on;
      |     
      |     subplot(3,1,2);
      |     plot(vect_wind_speed, lambda);
      |     axis([0, 35, 0, 20]);
      |     ylabel('Lambda');
      |     grid on;
      |     
      |     subplot(3,1,3)
      |     plot(vect_wind_speed, Cp);
      |     axis([0, 35, 0, .6]);
      |     xlabel('Wind Speed (m/s)');
      |     ylabel('Cp');
      |     set(gca,'ytick',[0 .1 .2 .3 .4 .5 .6]);
      |     grid on;
      | 
      |     hold off
      |     set_param(gcb,'DisplayTurbChar','off')
      |     
      | end
      mask TypeOptions ShowParameters: Generator data for 1 wind turbine | Converters data for 1 wind turbine | Turbine data for 1 wind turbine | Drive train data for 1 wind turbine | Control parameters for 1 wind turbine
      mask Callback ShowParameters:
      | BlockName=getfullname(gcb);
      | %
      | Param_Show=get_param(BlockName,'ShowParameters');
      | Param_DisplayTurbChar=get_param(BlockName,'DisplayTurbChar');
      | 
      | p_mask{3}='off';p_mask{4}='off';p_mask{5}='off';
      | p_mask{6}='off';p_mask{7}='off';p_mask{8}='off';p_mask{9}='off';
      | p_mask{10}='off';p_mask{11}='off';p_mask{12}='off';p_mask{13}='off';
      | p_mask{14}='off';p_mask{15}='off';p_mask{16}='off';p_mask{17}='off';
      | p_mask{18}='off';p_mask{19}='off';p_mask{20}='off';p_mask{21}='off';
      | p_mask{22}='off';p_mask{23}='off';p_mask{24}='off';p_mask{25}='off';
      | p_mask{26}='off';p_mask{27}='off';p_mask{28}='off';p_mask{29}='off';
      | p_mask{30}='off';p_mask{31}='off';p_mask{32}='off';p_mask{33}='off';
      | 
      | 
      | switch Param_Show
      | 	case 'Generator data for 1 wind turbine'
      | 		p_mask{3}='on';p_mask{4}='on';p_mask{5}='on'; p_mask{6}='on';
      |         p_mask{7}='on'; p_mask{8}='on';
      |     case 'Converters data for 1 wind turbine'
      | 		p_mask{9}='on';p_mask{10}='on';p_mask{11}='on';p_mask{12}='on';
      |         p_mask{13}='on';
      | 	case 'Turbine data for 1 wind turbine'
      |         p_mask{14}='on';p_mask{15}='on';p_mask{16}='on';p_mask{17}='on';
      |     case 'Drive train data for 1 wind turbine'
      |         p_mask{18}='on';p_mask{19}='on';p_mask{20}='on';p_mask{21}='on';
      |         p_mask{22}='on';
      |     case 'Control parameters for 1 wind turbine'
      |         p_mask{23}='on';p_mask{24}='on';p_mask{25}='on';
      |         p_mask{26}='on';p_mask{27}='on';p_mask{28}='on';p_mask{29}='on';
      |         p_mask{30}='on'; p_mask{31}='on';p_mask{32}='on'; p_mask{33}='on';
      | end
      | 
      | ParVisible={'on','on',p_mask{3},p_mask{4},p_mask{5},p_mask{6},p_mask{7},...
      |     p_mask{8},p_mask{9},p_mask{10},p_mask{11},p_mask{12},p_mask{13},...
      |     p_mask{14},p_mask{15},p_mask{16},p_mask{17},p_mask{18},p_mask{19},...
      |     p_mask{20},p_mask{21},p_mask{22},p_mask{23},p_mask{24},p_mask{25},...
      |     p_mask{26},p_mask{27},p_mask{28},p_mask{29},p_mask{30},p_mask{31},...
      |     p_mask{32},p_mask{33}};
      | %
      | set_param(BlockName,'MaskVisibilities',ParVisible);
      | set_param(BlockName,'DisplayTurbChar',Param_DisplayTurbChar);
  Demux : Demux  Outputs=2
  MW : Gain  Gain=37*2.1  SaturateOnIntegerOverflow=on  OutDataTypeStr=Inherit: Same as input  ParamDataTypeStr=Inherit: Same as input
  Mux : Mux  Inputs=2
  W1 (690 V) : spsThreePhaseVIMeasurementLib/Three-Phase V-I Measurement  VoltageMeasurement=phase-to-ground  SetLabelV=on  LabelV=Vabc_W1  Vpu=on  VpuLL=off  CurrentMeasurement=yes  SetLabelI=on  LabelI=Iabc_W1  Ipu=on  Pbase=37*2.1e6/0.9  Vbase=690  OutputType=Complex  PhasorSimulation=off  PSBequivalent=0
  Wind Farm Scope : Scope  NumInputPorts=6
  A : PMIOPort  Side=Left
  B : PMIOPort  Port=2  Side=Left
  C : PMIOPort  Port=3  Side=Left
  wires:
  [Vabc_W1] -> Wind Farm Scope/1  "Vabc_B575 (pu)"
  Demux/1 -> Wind Farm Scope/5  "P (MW)"
  Bus Selector/1 -> Wind Farm Scope/3  "<Vdc_V>"
  Demux/2 -> Wind Farm Scope/6  "Q (Mvar)"
  Mux/1 -> MW/1
  Bus Selector/2 -> Wind Farm Scope/4  "<wr_pu (IG speed)>"
  DFIG Wind Turbine/1(m) -> Bus Selector/1
  Bus Selector/3 -> Mux/1  "<P_pu>"
  Bus Selector/4 -> Mux/2  "<Q_pu>"
  MW/1 -> Demux/1
  [Iabc_W1] -> Wind Farm Scope/2  "Iabc_B575 (pu)"
  Constant2/1 -> DFIG Wind Turbine/1("Wind (m/s) ")
  Constant3/1 -> DFIG Wind Turbine/2(Qref_pu)
  connections:
  34.5 kV/ 690V 400 MVA/RConn2 -- W1 (690 V)/LConn2
  34.5 kV/ 690V 400 MVA/RConn1 -- W1 (690 V)/LConn1
  34.5 kV/ 690V 400 MVA/RConn3 -- W1 (690 V)/LConn3
  115 kV/34.5 kV 400 MVA/LConn1 -- 345kV/115 kV 400 MVA/RConn1
  115 kV/34.5 kV 400 MVA/LConn2 -- 345kV/115 kV 400 MVA/RConn2
  115 kV/34.5 kV 400 MVA/LConn3 -- 345kV/115 kV 400 MVA/RConn3
  34.5 kV/ 690V 400 MVA/LConn1 -- 1 km collector line/RConn1
  34.5 kV/ 690V 400 MVA/LConn2 -- 1 km collector line/RConn2
  34.5 kV/ 690V 400 MVA/LConn3 -- 1 km collector line/RConn3
  1 km collector line/LConn1 -- 115 kV/34.5 kV 400 MVA/RConn1
  1 km collector line/LConn2 -- 115 kV/34.5 kV 400 MVA/RConn2
  1 km collector line/LConn3 -- 115 kV/34.5 kV 400 MVA/RConn3
  W1 (690 V)/RConn1 -- DFIG Wind Turbine/LConn1
  W1 (690 V)/RConn2 -- DFIG Wind Turbine/LConn2
  W1 (690 V)/RConn3 -- DFIG Wind Turbine/LConn3
  345kV/115 kV 400 MVA/LConn2 -- B/RConn1
  345kV/115 kV 400 MVA/LConn1 -- A/RConn1
  345kV/115 kV 400 MVA/LConn3 -- C/RConn1
